simulink model "FlightControlSoftwareHardware"  (R2024a)
settings: Solver=FixedStepAuto  StartTime=0.0  StopTime=inf  RelTol=1e-3  EnableMultiTasking=on
PreLoadFcn:
  | load Data/PropData.mat;
undefined symbols (not defined in the file): DiscIntNeverNeededParam, PropData
libraries: arduinolib x1, slpidlib x1
settings Model: ExtModeTrigDuration=2  Creator=callie  LastModifiedBy=callie
settings SolverCC: AutoInsertRateTranBlk=on
settings OptimizationCC: EnhancedBackFolding=on  PassReuseOutputArgsAs=Individual arguments  ZeroExternalMemoryAtStartup=off  ZeroInternalMemoryAtStartup=off  MaxStackSize=64  OptimizeBlockOrder=speed  DifferentSizesBufferReuse=on  EfficientTunableParamExpr=on
settings DebuggingCC: ParameterTunabilityLossMsg=error
settings HardwareCC: ProdBitPerPointer=32  ProdBitPerSizeT=32  ProdBitPerPtrDiffT=32  ProdLargestAtomicInteger=Long  ProdLargestAtomicFloat=Double  ProdWordSize=32  ProdHWDeviceType=ARM Compatible->ARM Cortex
settings SFSimCC: MATLABDynamicMemAlloc=off
settings RTWCC: Description=Embedded Coder  SystemTargetFile=ert.tlc  HardwareBoard=Arduino Due  TemplateMakefile=ert_default_tmf  Toolchain=Arduino ARM  BuildConfiguration=Faster Runs
settings CodeAppCC: ForceParamTrailComments=on  IgnoreCustomStorageClasses=off  OperatorAnnotations=on  SimulinkDataObjDesc=on  SFDataObjDesc=on  InsertBlockDesc=on
settings ERTTargetCC: SupportContinuousTime=on  SupportVariableSizeSignals=on  ExtModeTransport=3  ExtModeStaticAlloc=on  ExtModeAutomaticAllocSize=off  ExtModeStaticAllocSize=24576  ExtModeMexFile=ext_xcp  ExtModeIntrfLevel=Level2 - Open

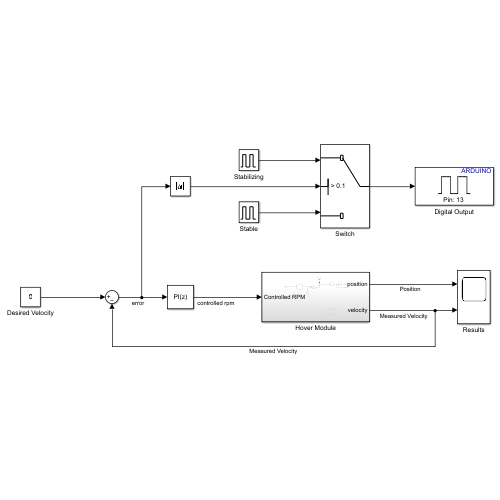
[thumbnail: Simulink's stored preview of the top-level diagram]
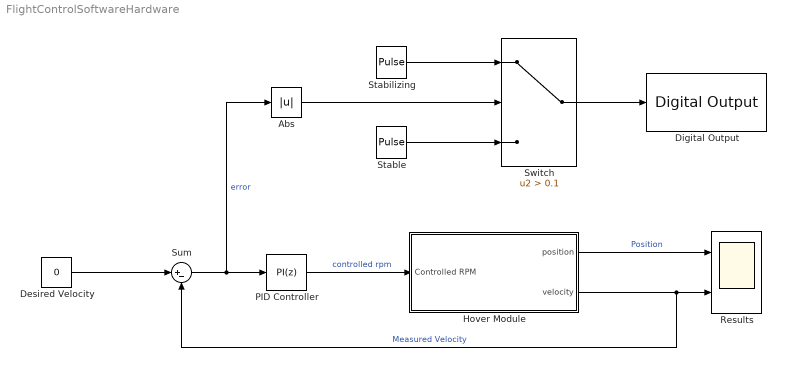
== system FlightControlSoftwareHardware ==
  Abs : Abs  SaturateOnIntegerOverflow=off
  Desired Velocity : Constant  Value=0  SampleTime=0.005
  Digital Output : arduinolib/Digital Output  pinNumber=13  Direction=output  blockPlatform=arduino
      settings: SourceProductName=Common
  Hover Module : Subsystem
  PID Controller : slpidlib/PID Controller  Controller=PI  Form=Parallel  TimeDomain=Discrete-time  UseExternalTs=off  SampleTime=-1  IntegratorMethod=Forward Euler  FilterMethod=Forward Euler  ControllerParametersSource=internal  P=10000  I=3500.0  UseKiTs=off  D=0  UseExternalDerivativeSource=off  N=100  UseFilter=on  TunerSelectOption=Transfer Function Based (PID Tuner App)  InitialConditionSource=internal  InitialConditionForIntegrator=0  InitialConditionForFilter=0  DifferentiatorICPrevScaledInput=0  ExternalReset=none  TrackingMode=off  Kt=1  LimitOutput=off  SatLimitsSource=internal  UpperSaturationLimit=inf  LowerSaturationLimit=-inf  LinearizeAsGain=on  AntiWindupMode=none  Kb=1  LimitIntegrator=off  UpperIntegratorSaturationLimit=inf  LowerIntegratorSaturationLimit=-inf  POutMin=[]  POutMax=[]  IOutMin=[]  IOutMax=[]  DOutMin=[]  DOutMax=[]  NOutMin=[]  NOutMax=[]  SumOutMin=[]  SumOutMax=[]  SaturationOutMin=[]  SaturationOutMax=[]  PParamMin=[]  PParamMax=[]  IParamMin=[]  IParamMax=[]  DParamMin=[]  DParamMax=[]  NParamMin=[]  NParamMax=[]  KbParamMin=[]  KbParamMax=[]  KtParamMin=[]  KtParamMax=[]  KbOutMin=[]  KbOutMax=[]  KtOutMin=[]  KtOutMax=[]  IntegratorOutMin=[]  IntegratorOutMax=[]  FilterOutMin=[]  FilterOutMax=[]  SumI1OutMin=[]  SumI1OutMax=[]  SumI2OutMin=[]  SumI2OutMax=[]  SumI3OutMin=[]  SumI3OutMax=[]  SumI4OutMin=[]  SumI4OutMax=[]  SumDOutMin=[]  SumDOutMax=[]  DifferentiatorOutMin=[]  DifferentiatorOutMax=[]  FilterDiffOutCoefMin=[]  FilterDiffOutCoefMax=[]  ReciprocalOutMin=[]  ReciprocalOutMax=[]  SumDenOutMin=[]  SumDenOutMax=[]  SumNumOutMin=[]  SumNumOutMax=[]  DivideOutMin=[]  DivideOutMax=[]  UdiffTsProdOutMin=[]  UdiffTsProdOutMax=[]  NTsProdOutMin=[]  NTsProdOutMax=[]  UintegralTsProdOutMin=[]  UintegralTsProdOutMax=[]  UngainTsProdOutMin=[]  UngainTsProdOutMax=[]  ClampingZeroOutDataTypeStr=Inherit: Inherit via back propagation  ClampingZeroOutMin=[]  ClampingZeroOutMax=[]  FilterDenConstantOutDataTypeStr=Inherit: Inherit via back propagation  FilterDenConstantOutMin=[]  FilterDenConstantOutMax=[]  PCopyOutDataTypeStr=Inherit: Inherit via back propagation  PCopyOutMin=[]  PCopyOutMax=[]  NCopyOutDataTypeStr=Inherit: Inherit via back propagation  NCopyOutMin=[]  NCopyOutMax=[]  IntegratorContinuousStateAttributes=''  IntegratorStateMustResolveToSignalObject=off  IntegratorRTWStateStorageClass=Auto  FilterContinuousStateAttributes=''  FilterStateMustResolveToSignalObject=off  FilterRTWStateStorageClass=Auto  ParallelPVariant=InternalParameters  IdealPVariant=Disabled  IVariant=InternalParameters  DVariant=Disabled  IntegratorVariant=Discrete  SatVariant=Disabled  AWVariant=Passthrough  PCopyVariant=Disabled  TRVariant=Disabled  FdbkBlocksVariant=Forward  IdealPFdbkVariant=Disabled  SatFdbkVariant=Disabled  DerivativeFilterVariant=Disabled  NVariant=Disabled  NCopyVariant=Disabled_SignalSpec  FilterICVariant=Disabled  IntegratorICVariant=InternalICs  ExternalResetVariant=Disabled  TRSumVariant=Passthrough  SumFdbkVariant=Disabled  SumVariant=Sum_PI  TsampFilterVariant=InternalTs  TsampNgainVariant=Passthrough  TsampIntegralVariant=Disabled_SignalSpec  ExternalSaturationOutDataTypeStr=Inherit: Same as second input  DerivativeSourceVariant=Disabled
  Results : Scope  NumInputPorts=2
  Stabilizing : DiscretePulseGenerator  PulseType=Time based  Period=0.2  PulseWidth=50
  Stable : DiscretePulseGenerator  PulseType=Time based  Period=0.5  PulseWidth=99
  Sum : Sum  Inputs=|+-
  Switch : Switch  Criteria=u2 > Threshold  Threshold=0.1  SaturateOnIntegerOverflow=off  InputSameDT=off
  wires:
  PID Controller/1 -> Hover Module/1(Controlled RPM)  "controlled rpm"
  Hover Module/1(position) -> Results/1  "Position"
  Sum/1 -> PID Controller/1, Abs/1  "error"
  Hover Module/2(velocity) -> Sum/2, Results/2  "Measured Velocity"
  Desired Velocity/1 -> Sum/1
  Stabilizing/1 -> Switch/1
  Switch/1 -> Digital Output/1
  Abs/1 -> Switch/2
  Stable/1 -> Switch/3

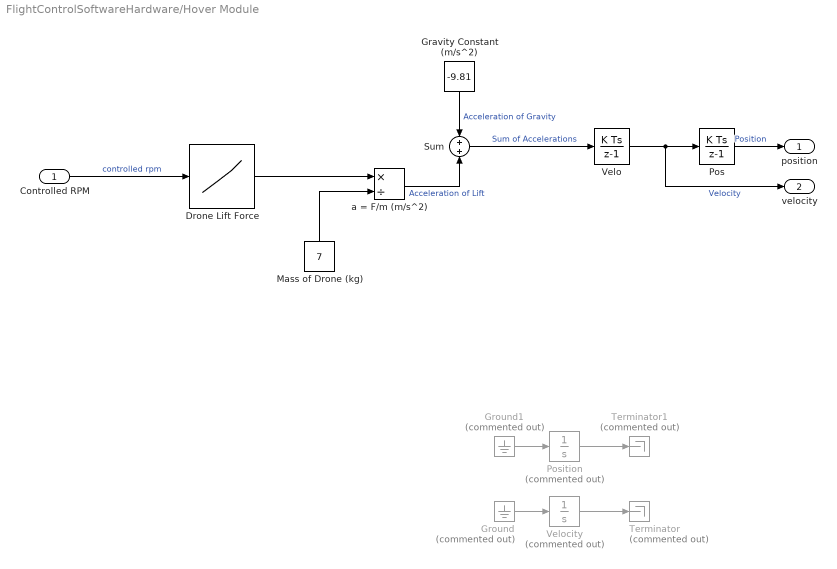
== system FlightControlSoftwareHardware/Hover Module ==
  Controlled RPM : Inport
  Drone Lift Force : Lookup_n-D  NumberOfTableDimensions=1  BreakpointsForDimension1=PropData.rpm  Table=PropData.lift  InternalRulePriority=Speed  RndMeth=Simplest
  Gravity Constant (m/s^2) : Constant  Value=-9.81
  Ground : Ground  Commented=on
  Ground1 : Ground  Commented=on
  Mass of Drone (kg) : Constant  Value=7
  Pos : DiscreteIntegrator  InitialCondition=15  SampleTime=-1  ICPrevOutput=DiscIntNeverNeededParam  ICPrevScaledInput=DiscIntNeverNeededParam
  Position : Integrator  Commented=on  InitialCondition=15
  Sum : Sum  Inputs=+|+
  Terminator : Terminator  Commented=on
  Terminator1 : Terminator  Commented=on
  Velo : DiscreteIntegrator  SampleTime=-1  ICPrevOutput=DiscIntNeverNeededParam  ICPrevScaledInput=DiscIntNeverNeededParam
  Velocity : Integrator  Commented=on
  a = F/m (m/s^2) : Product  Inputs=*/
  position : Outport  VectorParamsAs1DForOutWhenUnconnected=off
  velocity : Outport  Port=2  VectorParamsAs1DForOutWhenUnconnected=off
  wires:
  Controlled RPM/1 -> Drone Lift Force/1  "controlled rpm"
  Drone Lift Force/1 -> a = F/m (m/s^2)/1
  Velo/1 -> Pos/1, velocity/1  "Velocity"
  Sum/1 -> Velo/1  "Sum of Accelerations"
  Pos/1 -> position/1  "Position"
  a = F/m (m/s^2)/1 -> Sum/2  "Acceleration of Lift"
  Gravity Constant (m/s^2)/1 -> Sum/1  "Acceleration of Gravity"
  Mass of Drone (kg)/1 -> a = F/m (m/s^2)/2
  Velocity/1 -> Terminator/1
  Position/1 -> Terminator1/1
  Ground/1 -> Velocity/1
  Ground1/1 -> Position/1
